simulink model "Sl_LQR"  (R2015a)
settings: Solver=ode45  StartTime=0.0  StopTime=50  RelTol=1e-3
undefined symbols (not defined in the file): A, B, C, Kp, L
settings Model: Creator=Alex  LastModifiedBy=Vladislav

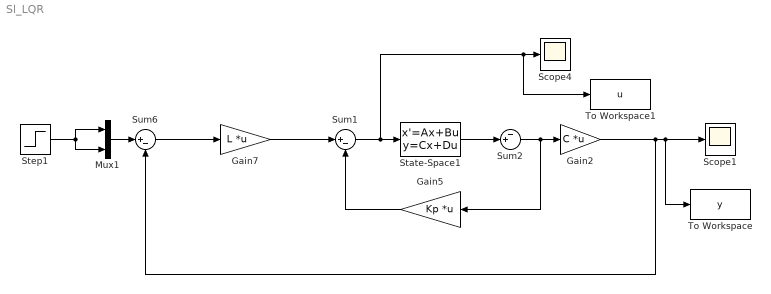
== system Sl_LQR ==
  Gain2 : Gain  Gain=C  Multiplication=Matrix(K*u)
  Gain5 : Gain  Gain=Kp  Multiplication=Matrix(K*u)
  Gain7 : Gain  Gain=L  Multiplication=Matrix(K*u)
  Mux1 : Mux  Inputs=2
  Scope1 : Scope
      settings: TimeRange=10  YMin=-0.2  YMax=1.2
  Scope4 : Scope
      settings: TimeRange=10  YMin=-0.2  YMax=1.4
  State-Space1 : StateSpace  A=A  B=B  C=eye(4)  D=zeros(4,2)  X0=0
  Step1 : Step  Time=0  After=2  SampleTime=0
  Sum1 : Sum  Inputs=|+-
  Sum2 : Sum  Inputs=-+|
  Sum6 : Sum  Inputs=|+-
  To Workspace : ToWorkspace  VariableName=y  SampleTime=-1
  To Workspace1 : ToWorkspace  VariableName=u  SampleTime=-1
  wires:
  Sum1/1 -> State-Space1/1, To Workspace1/1, Scope4/1
  Gain5/1 -> Sum1/2
  State-Space1/1 -> Sum2/2
  Sum2/1 -> Gain2/1, Gain5/1
  Gain7/1 -> Sum1/1
  Step1/1 -> Mux1/1, Mux1/2
  Mux1/1 -> Sum6/1
  Sum6/1 -> Gain7/1
  Gain2/1 -> To Workspace/1, Scope1/1, Sum6/2
